simulink model "A3Sim"  (R2017a)
settings: Solver=VariableStepAuto  StartTime=0.0  StopTime=inf  RelTol=1e-3
libraries: etargetslib x3, dspnetwork x3
settings Model: Creator=Ivan  LastModifiedBy=Ivan

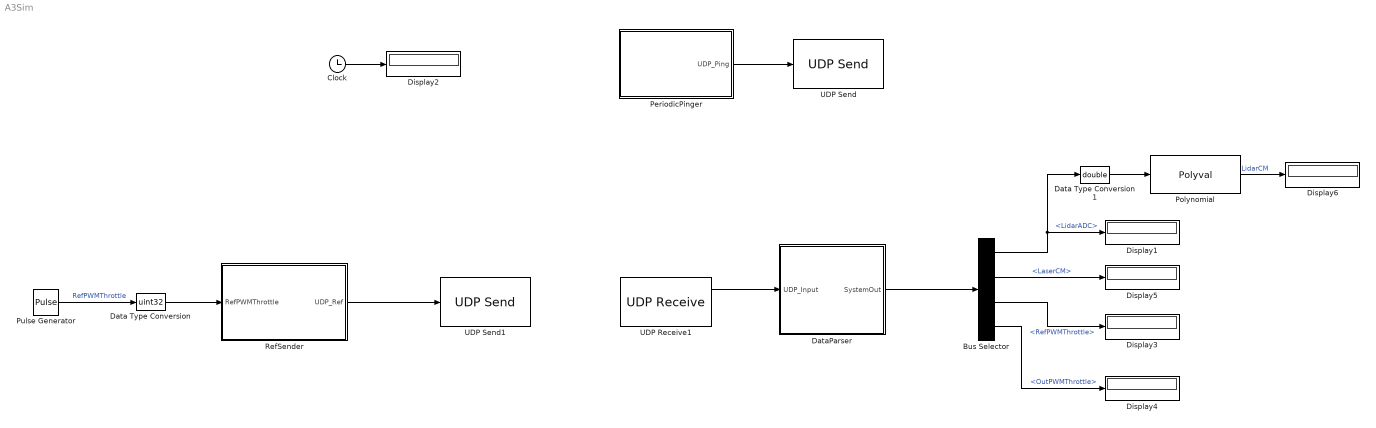
== system A3Sim ==
  Bus Selector : BusSelector  OutputSignals=LidarADC,LaserCM,RefPWMThrottle,OutPWMThrottle
  Clock : Clock
  Data Type Conversion : DataTypeConversion  OutDataTypeStr=uint32
  Data Type Conversion1 : DataTypeConversion  OutDataTypeStr=double
  DataParser : Subsystem
  Display{1..6} (6 alike) : Display
  PeriodicPinger : Subsystem
  Polynomial : Polyval  Coefs=[-7.999269172741439e-07,0.001591223144821,-1.090589949213111,2.816298617557626e+02]
  Pulse Generator : DiscretePulseGenerator  PulseType=Time based  Amplitude=100  Period=1  PulseWidth=50
  RefSender : Subsystem
  UDP Receive1 : dspnetwork/UDP Receive  localURL='0.0.0.0'  localPort=25000  remoteURL='0.0.0.0'  remotePort=-1  recvBufferSize=8192  dims=31  signalDatatype=uint8  isVarSize=off  showBlockingTime=on  blockingTime=0.1  sampletime=0.02  blockPlatform=HOST
  UDP Send : dspnetwork/UDP Send  remoteURL='192.168.0.121'  remotePort=12000  localURL='0.0.0.0'  localPortSource=Automatically determine  localPort=-1  sampletime=-1  blockPlatform=HOST  separateLengthPort=0
  UDP Send1 : dspnetwork/UDP Send  remoteURL='192.168.0.121'  remotePort=12000  localURL='0.0.0.0'  localPortSource=Automatically determine  localPort=-1  sampletime=-1  blockPlatform=HOST  separateLengthPort=0
  wires:
  Clock/1 -> Display2/1
  PeriodicPinger/1(UDP_Ping) -> UDP Send/1
  Bus Selector/1 -> Data Type Conversion1/1, Display1/1  "<LidarADC>"
  Bus Selector/2 -> Display5/1  "<LaserCM>"
  UDP Receive1/1 -> DataParser/1(UDP_Input)
  DataParser/1(SystemOut) -> Bus Selector/1
  Bus Selector/3 -> Display3/1  "<RefPWMThrottle>"
  Pulse Generator/1 -> Data Type Conversion/1  "RefPWMThrottle"
  RefSender/1(UDP_Ref) -> UDP Send1/1
  Data Type Conversion/1 -> RefSender/1(RefPWMThrottle)
  Bus Selector/4 -> Display4/1  "<OutPWMThrottle>"
  Polynomial/1 -> Display6/1  "LidarCM"
  Data Type Conversion1/1 -> Polynomial/1

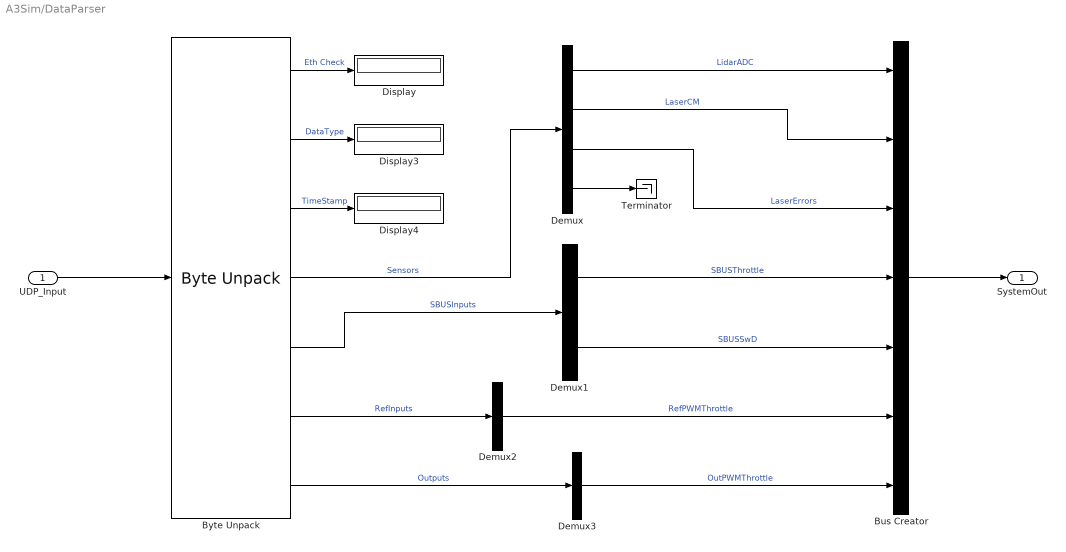
== system A3Sim/DataParser ==
  UDP_Input : Inport
  Bus Creator : BusCreator  Inputs=7
  Byte Unpack : etargetslib/Byte Unpack  dimensions={[2],[1],[1],[4],[2],[1],[1]}  datatypes={'uint8','uint8','uint32', 'uint16', 'uint32', 'uint32', 'uint32'}  byteAlign=1
  Demux : Demux
  Demux1 : Demux  Outputs=2
  Demux2 : Demux  Outputs=1
  Demux3 : Demux  Outputs=1
  Display : Display
  Display3 : Display
  Display4 : Display
  Terminator : Terminator
  SystemOut : Outport
  wires:
  UDP_Input/1 -> Byte Unpack/1
  Demux1/2 -> Bus Creator/5  "SBUSSwD"
  Byte Unpack/7 -> Demux3/1  "Outputs"
  Byte Unpack/4 -> Demux/1  "Sensors"
  Byte Unpack/1 -> Display/1  "Eth Check"
  Demux/4 -> Terminator/1
  Demux/3 -> Bus Creator/3  "LaserErrors"
  Demux3/1 -> Bus Creator/7  "OutPWMThrottle"
  Byte Unpack/3 -> Display4/1  "TimeStamp"
  Demux/2 -> Bus Creator/2  "LaserCM"
  Demux/1 -> Bus Creator/1  "LidarADC"
  Bus Creator/1 -> SystemOut/1
  Byte Unpack/6 -> Demux2/1  "RefInputs"
  Byte Unpack/2 -> Display3/1  "DataType"
  Byte Unpack/5 -> Demux1/1  "SBUSInputs"
  Demux2/1 -> Bus Creator/6  "RefPWMThrottle"
  Demux1/1 -> Bus Creator/4  "SBUSThrottle"

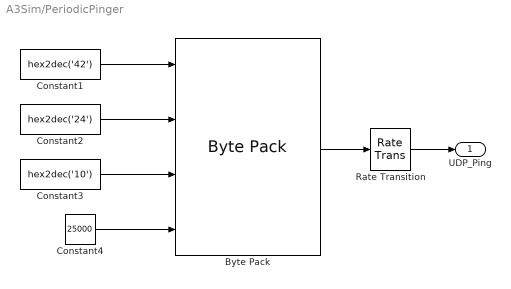
== system A3Sim/PeriodicPinger ==
  Byte Pack : etargetslib/Byte Pack  datatypes={'uint8','uint8','uint8','uint16'}  byteAlign=1
  Constant1 : Constant  Value=hex2dec('42')  OutDataTypeStr=uint8
  Constant2 : Constant  Value=hex2dec('24')  OutDataTypeStr=uint8
  Constant3 : Constant  Value=hex2dec('10')  OutDataTypeStr=uint8
  Constant4 : Constant  Value=25000  OutDataTypeStr=uint16
  Rate Transition : RateTransition  OutPortSampleTime=1
  UDP_Ping : Outport
  wires:
  Constant3/1 -> Byte Pack/3
  Byte Pack/1 -> Rate Transition/1
  Constant1/1 -> Byte Pack/1
  Constant2/1 -> Byte Pack/2
  Constant4/1 -> Byte Pack/4
  Rate Transition/1 -> UDP_Ping/1

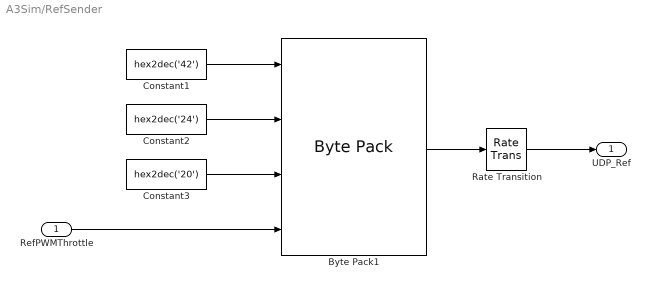
== system A3Sim/RefSender ==
  RefPWMThrottle : Inport
  Byte Pack1 : etargetslib/Byte Pack  datatypes={'uint8','uint8','uint8','uint32'}  byteAlign=1
  Constant1 : Constant  Value=hex2dec('42')  OutDataTypeStr=uint8
  Constant2 : Constant  Value=hex2dec('24')  OutDataTypeStr=uint8
  Constant3 : Constant  Value=hex2dec('20')  OutDataTypeStr=uint8
  Rate Transition : RateTransition  OutPortSampleTime=0.02
  UDP_Ref : Outport
  wires:
  Byte Pack1/1 -> Rate Transition/1
  Rate Transition/1 -> UDP_Ref/1
  RefPWMThrottle/1 -> Byte Pack1/4
  Constant1/1 -> Byte Pack1/1
  Constant3/1 -> Byte Pack1/3
  Constant2/1 -> Byte Pack1/2
